simulink model "Earthquake_Stabilizer"  (R2015b)
settings: Solver=FixedStepDiscrete  StartTime=0.0  StopTime=inf  FixedStep=0.002  RelTol=1e-3
undefined symbols (not defined in the file): HIL, qc_get_step_size, serial
libraries: quarc_library x6, instrumentlib x2, simulink x1
settings Model: SimulationMode=external  ExtModeTrigDuration=5000  Creator=REACH_1  LastModifiedBy=jtill
settings SolverCC: PositivePriorityOrder=on
settings RTWCC: SystemTargetFile=quarc_win64.tlc  TemplateMakefile=quarc_default_tmf  Description=QUARC Win64 Target
settings STFCustomTargetCC: GeneratePreprocessorConditionals=Use local settings  CPPClassGenCompliant=off
settings GRTTargetCC: ParMdlRefBuildCompliant=off  CompOptLevelCompliant=off  CombineOutputUpdateFcns=off  MatFileLogging=off  CPPClassGenCompliant=off  GRTInterface=on  UseToolchainInfoCompliant=off  ExtMode=on  ExtModeMexFile=quarc_comm

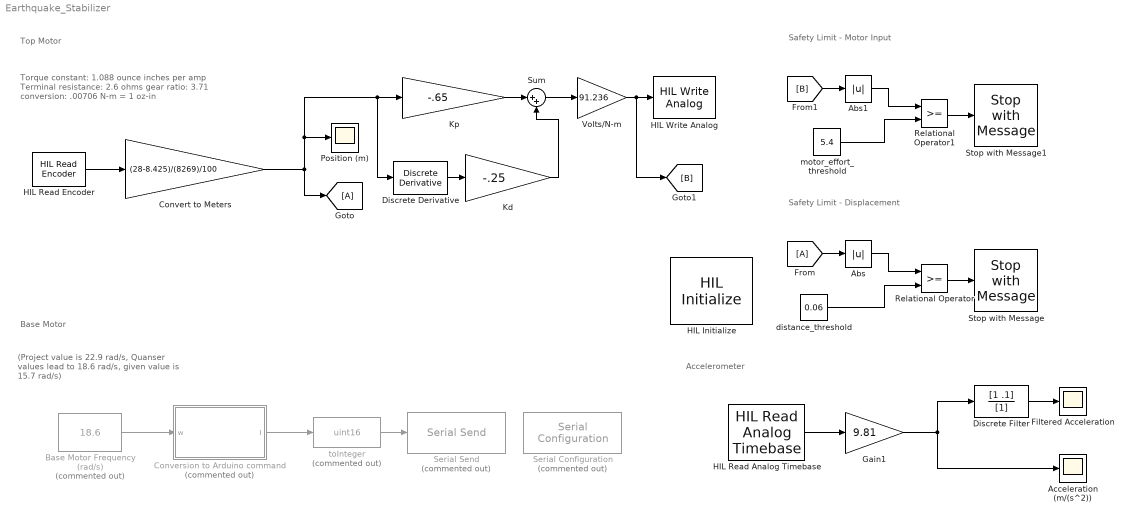
== system Earthquake_Stabilizer ==
  note: (Project value is 22.9 rad/s,
      |  Quanser values lead to 18.6 rad/s,
      |   given value is 15.7 rad/s)
  note: Safety Limit - Displacement
  note: Top Motor
  note: Accelerometer
  note: Base Motor
  note: Torque constant: 1.088 ounce inches per amp
      | Terminal resistance: 2.6 ohms
      | gear ratio: 3.71
      | conversion: .00706 N-m = 1 oz-in
  note: Safety Limit - Motor Input
  Abs : Abs
  Abs1 : Abs
  Acceleration (m/(s^2)) : Scope
  Base Motor Frequency (rad/s) : Constant  Commented=on  Value=18.6  SampleTime=3
  Conversion to Arduino command : MATLAB Function  Commented=on  TreatAsAtomicUnit=on
  Convert to Meters : Gain  Gain=(28-8.425)/(8269)/100
  Discrete Derivative : simulink/Discrete/Discrete Derivative  gainval=1.0  ICPrevScaledInput=0.0  InputProcessing=Inherited  OutMin=[]  OutMax=[]  OutDataType=fixdt(1, 16)  OutScaling=2^-10  DoSatur=off
  Discrete Filter : DiscreteFilter  Numerator=[1 .1]  Denominator=[1]
  Filtered Acceleration : Scope
  Gain1 : Gain  Gain=9.81
  HIL Initialize : quarc_library/Data Acquisition/Generic/Configuration/HIL Initialize  Priority=-99  object_name=HIL-1  board_type=q2_usb  board_number=0  board_options=d0=digital;d1=digital;led=auto;update_rate=normal;decimation=1  exclusive=off  active=off  hardware_clocks=[0]  clock_modes=[]  initial_clock_frequencies=[]  set_clock_params_at_start=off  set_clock_params_at_switch_in=off  set_clock_frequencies_at_start=off  set_clock_frequencies_at_switch_in=off  analog_input_channels=[0:1]  analog_input_maximums=10  analog_input_minimums=-10  set_analog_input_params_at_start=on  set_analog_input_params_at_switch_in=off  analog_output_channels=[0:1]  analog_output_maximums=10  analog_output_minimums=-10  initial_analog_outputs=[0]  final_analog_outputs=[0]  watchdog_analog_outputs=0  set_analog_output_params_at_start=on  set_analog_output_params_at_switch_in=off  set_analog_outputs_at_start=on  set_analog_outputs_at_switch_in=off  set_analog_outputs_at_terminate=on  set_analog_outputs_at_switch_out=off  set_analog_outputs_on_watchdog=off  digital_input_channels=[]  digital_output_channels=[]  digital_output_configuration=[]  initial_digital_outputs=[1]  final_digital_outputs=[1]  watchdog_digital_outputs=[1]  set_digital_output_params_at_start=off  set_digital_output_params_at_switch_in=off  set_digital_outputs_at_start=on  set_digital_outputs_at_switch_in=off  set_digital_outputs_at_terminate=on  set_digital_outputs_at_switch_out=off  set_digital_outputs_on_watchdog=off  encoder_channels=[0:1]  quadrature=[4]  encoder_filter_frequency=[]  initial_encoder_counts=[0]  set_encoder_params_at_start=on  set_encoder_params_at_switch_in=off  set_encoder_counts_at_start=on  set_encoder_counts_at_switch_in=off  pwm_channels=[]  pwm_modes=[0]  pwm_frequency=1/0.020  pwm_configuration=[]  pwm_alignment=[]  pwm_polarity=[]  pwm_leading_deadband=[]  pwm_trailing_deadband=[]  initial_pwm_outputs=[0]  final_pwm_outputs=[0]  watchdog_pwm_outputs=[0]  set_pwm_params_at_start=on  set_pwm_params_at_switch_in=off  set_pwm_outputs_at_start=on  set_pwm_outputs_at_switch_in=off  set_pwm_outputs_at_terminate=on  set_pwm_outputs_at_switch_out=off  set_pwm_outputs_on_watchdog=off  other_output_channels=[]  initial_other_outputs=[]  final_other_outputs=[]  watchdog_other_outputs=[]  set_other_outputs_at_start=off  set_other_outputs_at_switch_in=off  set_other_outputs_at_terminate=off  set_other_outputs_at_switch_out=off  set_other_outputs_on_watchdog=off
  HIL Read Analog Timebase : quarc_library/Data Acquisition/Generic/Timebases/HIL Read Analog Timebase  object_name=HIL-1  clock=0  channels=0  samples_in_buffer=max(ceil(1/qc_get_step_size), 1)  active=on  vector_output=off
      settings: AttributesFormatString=(%<object_name>)
  HIL Read Encoder : quarc_library/Data Acquisition/Generic/Immediate I//O/HIL Read Encoder  object_name=HIL-1  channels=0  sample_time=qc_get_step_size  active=on  vector_output=off  data_type_mode=Inherit via back propagation  data_type=double
  HIL Write Analog : quarc_library/Data Acquisition/Generic/Immediate I//O/HIL Write Analog  object_name=HIL-1  channels=0  sample_time=-1  active=off  vector_input=off
  Kd : Gain  Gain=-.25
  Kp : Gain  Gain=-.65
  "Position (m) " : Scope
  Relational Operator : RelationalOperator  OutDataTypeStr=boolean
  Relational Operator1 : RelationalOperator  OutDataTypeStr=boolean
  Serial Configuration : instrumentlib/Serial Configuration  Priority=-200000  Commented=on  ComPortMenu=<Please select a port...>  ComPort=COM8  ObjConstructor=serial('COM8');  BaudRate=9600  DataBits=8  Parity=none  StopBits=1  FlowControl=none  Timeout=1000  ByteOrder=LittleEndian
  Serial Send : instrumentlib/Serial Send  Commented=on  ComPortMenu=<Please select a port...>  ComPort=COM8  ObjConstructor=serial('COM8');  Terminator=<none>  EnableBlockingMode=on
  Stop with Message : quarc_library/Sinks/Error Handling/Stop with Message  message_type=Fixed error message  message_icon=Error  message=TERMINATED - Encroaching on displacement safety limits
  Stop with Message1 : quarc_library/Sinks/Error Handling/Stop with Message  message_type=Fixed error message  message_icon=Error  message=TERMINATED - Encroaching on motor effort safety limits
  Sum : Sum  Inputs=|++
  Volts/N-m : Gain  Gain=91.236
  distance_threshold : Constant  Value=0.06
  motor_effort_threshold : Constant  Value=5.4
  toInteger : DataTypeConversion  Commented=on  OutDataTypeStr=uint16  RndMeth=Nearest
  wires:
  HIL Read Analog Timebase/1 -> Gain1/1
  HIL Read Encoder/1 -> Convert to Meters/1
  Convert to Meters/1 -> Kp/1, Discrete Derivative/1, "Position (m) "/1, [A]
  Gain1/1 -> Acceleration (m/(s^2))/1, Discrete Filter/1
  Abs/1 -> Relational Operator/1
  distance_threshold/1 -> Relational Operator/2
  Relational Operator/1 -> Stop with Message/1
  Discrete Derivative/1 -> Kd/1
  Kp/1 -> Sum/1
  Kd/1 -> Sum/2
  Sum/1 -> Volts/N-m/1
  Volts/N-m/1 -> [B], HIL Write Analog/1
  Base Motor Frequency (rad/s)/1 -> Conversion to Arduino command/1(w)
  [A] -> Abs/1
  toInteger/1 -> Serial Send/1
  Conversion to Arduino command/1(I) -> toInteger/1
  Discrete Filter/1 -> Filtered Acceleration/1
  Abs1/1 -> Relational Operator1/1
  motor_effort_threshold/1 -> Relational Operator1/2
  Relational Operator1/1 -> Stop with Message1/1
  [B] -> Abs1/1

== matlab function Earthquake_Stabilizer/Conversion to Arduino command ==
  data: w input; I output
function I = RadPerSec2Integer(w)
%#codegen

rpm_max = 251;
f_max = rpm_max/60;
w_max = 2*pi*f_max;

I = round( w/w_max * 255 );
